simulink model "problem53"  (Simulink 10.1)
settings: Solver=FixedStepAuto  StartTime=0.0  StopTime=100  FixedStep=0.001  RelTol=1e-6  EnableMultiTasking=on
values from neighbouring files (symbols this model uses):
  I = [Ixx 0 0; 0 1.9*Ixx 0; 0 0 Izz]    [main.m]
  invI = I^-1    [main.m]
  Q0 = [Q0S Q0V]    [main.m]
  w0 = [0; 5; 30]*pi/180    [main.m]
libraries: Quat2Euler x1
settings Model: Creator=eess  LastModifiedBy=Laura
settings DataIOCC: LimitDataPoints=on  SignalLoggingSaveFormat=ModelDataLogs
settings OptimizationCC: ExpressionDepthLimit=2147483647
settings DebuggingCC: SolverPrmCheckMsg=warning  FcnCallInpInsideContextMsg=warning  StateNameClashWarn=warning
settings ConfigComp: CovHtmlReporting=off

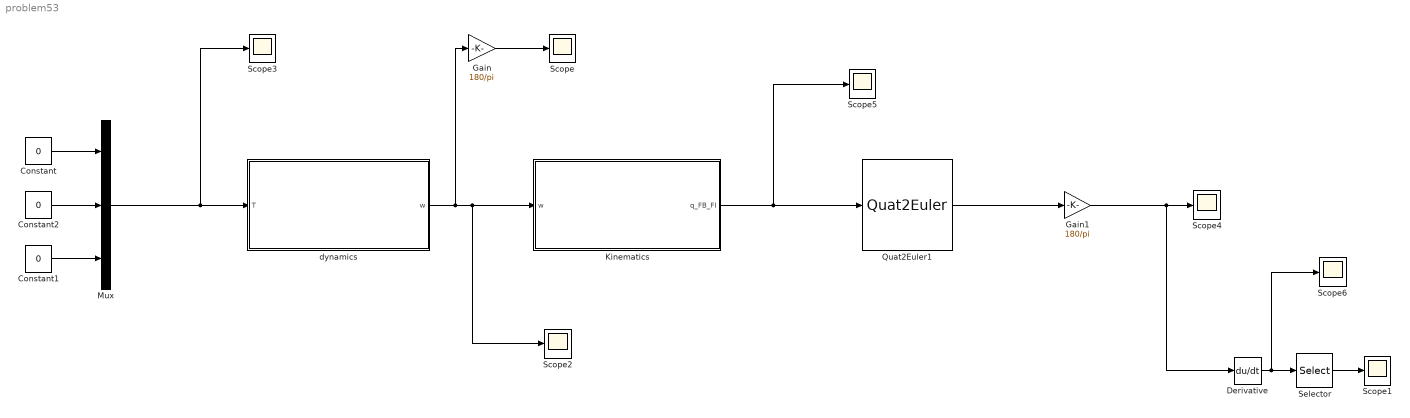
== system problem53 ==
  Constant : Constant  Value=0
  Constant1 : Constant  Value=0
  Constant2 : Constant  Value=0
  Derivative : Derivative
  Gain : Gain  Gain=180/pi
  Gain1 : Gain  Gain=180/pi
  Kinematics : Subsystem
  Mux : Mux  Inputs=3
  Quat2Euler1 : Quat2Euler/Quat2Euler  euler_order=313  quat_convention=1
  Scope{,1..6} (7 alike) : Scope
  Selector : Selector  InputPortWidth=3  IndexOptions=Index vector (dialog)  Indices=[1]  OutputSizes=1
  dynamics : Subsystem
  wires:
  dynamics/1(w) -> Gain/1, Scope2/1, Kinematics/1(w)
  Kinematics/1(q_FB_FI) -> Quat2Euler1/1, Scope5/1
  Quat2Euler1/1 -> Gain1/1
  Derivative/1 -> Scope6/1, Selector/1
  Selector/1 -> Scope1/1
  Constant/1 -> Mux/1
  Constant1/1 -> Mux/3
  Mux/1 -> Scope3/1, dynamics/1(T)
  Gain1/1 -> Scope4/1, Derivative/1
  Gain/1 -> Scope/1
  Constant2/1 -> Mux/2

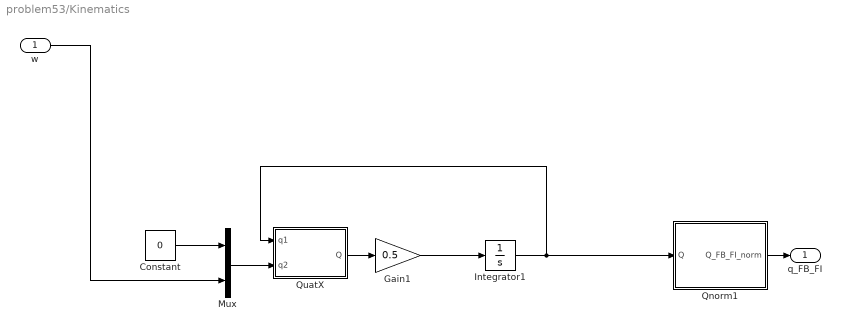
== system problem53/Kinematics ==
  w : Inport
  Constant : Constant  Value=0
  Gain1 : Gain  Gain=0.5
  Integrator1 : Integrator  InitialCondition=Q0
  Mux : Mux  Inputs=2
  Qnorm1 : Subsystem
  QuatX : MATLAB Function  TreatAsAtomicUnit=on
  q_FB_FI : Outport  VectorParamsAs1DForOutWhenUnconnected=off
  wires:
  w/1 -> Mux/2
  QuatX/1(Q) -> Gain1/1
  Gain1/1 -> Integrator1/1
  Integrator1/1 -> QuatX/1(q1), Qnorm1/1(Q)
  Constant/1 -> Mux/1
  Mux/1 -> QuatX/2(q2)
  Qnorm1/1(Q_FB_FI_norm) -> q_FB_FI/1

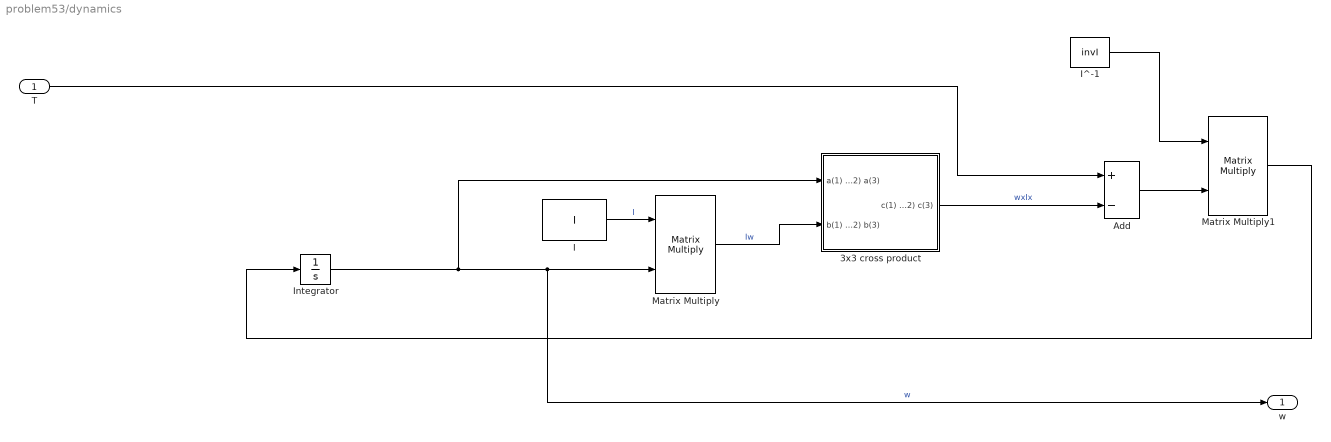
== system problem53/dynamics ==
  T : Inport
  3x3 cross product : Subsystem  AncestorBlock=cross1/3x3 cross product  mask(Cross Product){}
      mask help: Cross Product
      mask Help: eval( 'shelp sbcross1' );
      mask Display:
      | disp('Cross\nC=AXB')
      | port_label('input',1,'A')
      | port_label('input',2,'B')
      | port_label('output',1,'C')
  Add : Sum  Inputs=+-
  I : Constant  Value=I
  I^-1 : Constant  Value=invI
  Integrator : Integrator  InitialCondition=w0
  Matrix Multiply : Product  Multiplication=Matrix(*)
  Matrix Multiply1 : Product  Multiplication=Matrix(*)
  w : Outport  VectorParamsAs1DForOutWhenUnconnected=off
  wires:
  I/1 -> Matrix Multiply/1  "I"
  Integrator/1 -> 3x3 cross product/1(a(1) a(2) a(3)), Matrix Multiply/2, w/1  "w"
  Matrix Multiply/1 -> 3x3 cross product/2(b(1) b(2) b(3))  "Iw"
  Add/1 -> Matrix Multiply1/2
  I^-1/1 -> Matrix Multiply1/1
  Matrix Multiply1/1 -> Integrator/1
  3x3 cross product/1(c(1) c(2) c(3)) -> Add/2  "wxIx"
  T/1 -> Add/1

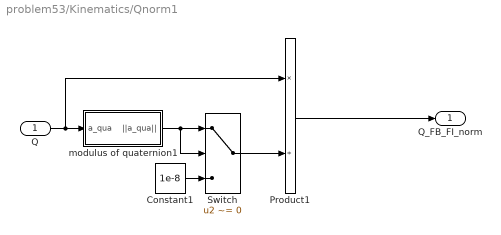
== system problem53/Kinematics/Qnorm1 ==
  Q : Inport
  Constant1 : Constant  Value=1e-8  SampleTime=-1
  Product1 : Product  Inputs=*/  InputSameDT=on  RndMeth=Zero  SaturateOnIntegerOverflow=on  OutDataTypeStr=Inherit: Same as first input
  Switch : Switch  Criteria=u2 ~= 0
  modulus of quaternion1 : Subsystem
      settings: AttributesFormatString=modulus of quaternion
  Q_FB_FI_norm : Outport  VectorParamsAs1DForOutWhenUnconnected=off
  wires:
  Q/1 -> Product1/1, modulus of quaternion1/1(a_qua)
  Switch/1 -> Product1/2
  Constant1/1 -> Switch/3
  modulus of quaternion1/1(||a_qua||) -> Switch/1, Switch/2
  Product1/1 -> Q_FB_FI_norm/1

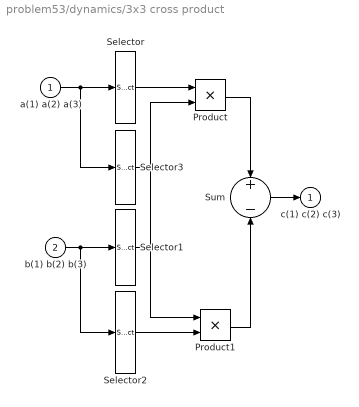
== system problem53/dynamics/3x3 cross product ==
  a(1) a(2) a(3) : Inport
  b(1) b(2) b(3) : Inport  Port=2
  Product : Product  InputSameDT=on  RndMeth=Zero  SaturateOnIntegerOverflow=on  OutDataTypeStr=Inherit: Same as first input
  Product1 : Product  InputSameDT=on  RndMeth=Zero  SaturateOnIntegerOverflow=on  OutDataTypeStr=Inherit: Same as first input
  Selector : Selector  InputPortWidth=3  IndexOptions=Index vector (dialog)  Indices=[2 3 1]  OutputSizes=1
  Selector1 : Selector  InputPortWidth=3  IndexOptions=Index vector (dialog)  Indices=[3 1 2]  OutputSizes=1
  Selector2 : Selector  InputPortWidth=3  IndexOptions=Index vector (dialog)  Indices=[2 3 1]  OutputSizes=1
  Selector3 : Selector  InputPortWidth=3  IndexOptions=Index vector (dialog)  Indices=[3 1 2]  OutputSizes=1
  Sum : Sum  Inputs=+|-  InputSameDT=on  SaturateOnIntegerOverflow=on  OutDataTypeStr=Inherit: Same as first input
  c(1) c(2) c(3) : Outport  InitialOutput=0  VectorParamsAs1DForOutWhenUnconnected=off
  wires:
  Selector3/1 -> Product1/1
  Selector2/1 -> Product1/2
  Product1/1 -> Sum/2
  Selector1/1 -> Product/2
  Product/1 -> Sum/1
  a(1) a(2) a(3)/1 -> Selector3/1, Selector/1
  Selector/1 -> Product/1
  b(1) b(2) b(3)/1 -> Selector2/1, Selector1/1
  Sum/1 -> c(1) c(2) c(3)/1

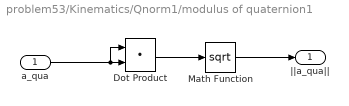
== system problem53/Kinematics/Qnorm1/modulus of quaternion1 ==
  a_qua : Inport
  Dot Product : DotProduct  InputSameDT=on  OutDataTypeStr=Inherit: Inherit via internal rule
  Math Function : Math  Operator=sqrt  SignedPower=on  SaturateOnIntegerOverflow=on
  ||a_qua|| : Outport  VectorParamsAs1DForOutWhenUnconnected=off
  wires:
  a_qua/1 -> Dot Product/2, Dot Product/1
  Math Function/1 -> ||a_qua||/1
  Dot Product/1 -> Math Function/1

== matlab function Kinematics/QuatX ==
  data: q1 input double; Q output double; q2 input double
function Q = fcn(q1,q2)
% This function performs the quaternions multiplication
%
q10 = q1(1);
q1v = q1(2:4);
%
q20 = q2(1);
q2v = q2(2:4);
%
Q0 = q10*q20 - dot(q1v, q2v);
Qv = q10*q2v + q20*q1v + cross(q1v,q2v);
%
Q = [Q0;Qv];
